simulink model "e03_MtrCtrl_MtrCtrl"  (R2024a)
settings: Solver=FixedStepDiscrete  StartTime=0.0  StopTime=1  FixedStep=mSim.dTime  MaxStep=Define.sModelSampleTime  RelTol=7.1420e-05
undefined symbols (not defined in the file): CnstCnst, CnstMde, CnstNr, E03CCTRL, E03INIT, E03LIM, E03MCMV, sTempGain
libraries: Lib_LPF x2
(part 1 of 3)
settings Model: Creator=user  LastModifiedBy=admin
settings SolverCC: MaxConsecutiveZCs=10000  ZeroCrossAlgorithm=Adaptive  AlgebraicLoopSolver=TrustRegion
settings DataIOCC: SaveOutput=off  DSMLogging=off  InspectSignalLogs=on  SaveTime=off  SignalLoggingName=logsout_Validator
settings OptimizationCC: BlockReduction=off  DefaultParameterBehavior=Inlined  UseDivisionForNetSlopeComputation=UseDivisionForReciprocalsOfIntegersOnly  GainParamInheritBuiltInType=on  UseFloatMulNetSlope=on  DefaultUnderspecifiedDataType=single  InlineInvariantSignals=on  BitwiseOrLogicalOp=Logical operator  PassReuseOutputArgsAs=Individual arguments  EfficientFloat2IntCast=on  LifeSpan=Inf  OptimizeBlockOrder=speed  DifferentSizesBufferReuse=on  EfficientTunableParamExpr=on
settings DebuggingCC: SignalInfNanChecking=error  SignalRangeChecking=error  ReadBeforeWriteMsg=EnableAllAsError  WriteAfterWriteMsg=EnableAllAsError  WriteAfterReadMsg=EnableAllAsError  AlgebraicLoopMsg=error  ArtificialAlgebraicLoopMsg=error  SaveWithDisabledLinksMsg=error  SaveWithParameterizedLinksMsg=error  BlockPriorityViolationMsg=error  SolverPrmCheckMsg=error  InheritedTsInSrcMsg=error  SingleTaskRateTransMsg=error  TasksWithSamePriorityMsg=error  SigSpecEnsureSampleTimeMsg=error  CheckMatrixSingularityMsg=error  IntegerOverflowMsg=error  ParameterUnderflowMsg=error  ParameterPrecisionLossMsg=error  ParameterTunabilityLossMsg=error  UnderSpecifiedDataTypeMsg=error  UnnecessaryDatatypeConvMsg=warning  VectorMatrixConversionMsg=error  SignalLabelMismatchMsg=error  UnconnectedInputMsg=error  UnconnectedOutputMsg=error  UnconnectedLineMsg=error  SFcnCompatibilityMsg=error  UniqueDataStoreMsg=error  BusObjectLabelMismatch=error  RootOutportRequireBusObject=error  AssertControl=DisableAll  ModelReferenceIOMismatchMessage=error  UnknownTsInhSupMsg=error  ModelReferenceDataLoggingMessage=error  ModelReferenceSymbolNameMessage=none  StateNameClashWarn=warning  StrictBusMsg=ErrorOnBusTreatedAsVector  NonBusSignalsTreatedAsBus=error  SFInvalidInputDataAccessInChartInitDiag=error  SFTransitionOutsideNaturalParentDiag=error  SFUnreachableExecutionPathDiag=error  SFUndirectedBroadcastEventsDiag=error  SFTransitionActionBeforeConditionDiag=error  SFTemporalDelaySmallerThanSampleTimeDiag=error  SFSelfTransitionDiag=error  SFExecutionAtInitializationDiag=error  IntegerSaturationMsg=error  UnitsInconsistencyMsg=none  VariantConditionMismatch=error
settings HardwareCC: ProdBitPerChar=16  ProdBitPerInt=16  ProdBitPerPointer=32  ProdBitPerSizeT=32  ProdBitPerPtrDiffT=32  ProdLargestAtomicInteger=Integer  ProdLargestAtomicFloat=None  ProdWordSize=16  ProdLongLongMode=on  ProdHWDeviceType=Texas Instruments->C2000
settings ModelReferenceCC: EnableRefExpFcnMdlSchedulingChecks=on  ModelReferenceNumInstancesAllowed=Single
settings SFSimCC: SimUseLocalCustomCode=off  CompileTimeRecursionLimit=0  EnableRuntimeRecursion=off  MATLABDynamicMemAlloc=off  CustomCodeUndefinedFunction=UseInterfaceOnly
settings RTWCC: Description=Embedded Coder  SystemTargetFile=ert.tlc  GenCodeOnly=on  TemplateMakefile=ert_default_tmf  GenerateReport=on  RTWUseLocalCustomCode=off  BuildConfiguration=Faster Runs  IncludeHyperlinkInReport=on  LaunchReport=on  GenerateTraceInfo=on  GenerateTraceReport=on  GenerateTraceReportSl=on  GenerateTraceReportSf=on  GenerateWebview=on  GenerateCodeMetricsReport=on  GenerateCodeReplacementReport=on  GPUComputeCapability=3.5  DLArmComputeVersion=19.05
settings CodeAppCC: ForceParamTrailComments=on  IgnoreCustomStorageClasses=off  MATLABFcnDesc=on  MangleLength=4  CustomSymbolStrGlobalVar=GvE03$N$M  CustomSymbolStrType=StrE03$N$M  CustomSymbolStrFcn=$N$M$F  CustomSymbolStrMacro=$N$M  DefineNamingRule=UpperCase  ParamNamingRule=UpperCase  SimulinkBlockComments=off  MATLABSourceComments=on  EnableCustomComments=on  ReqsInCode=on
settings ERTTargetCC: TargetLangStandard=C99 (ISO)  UtilityFuncGeneration=Shared location  MultiwordLength=2048  IncludeMdlTerminateFcn=off  CombineSignalStateStructs=on  SuppressErrorStatus=on  SupportAbsoluteTime=off  SupportNonFinite=off  ParenthesesLevel=Maximum  CastingMode=Standards  GenerateSharedConstants=off  InlinedParameterPlacement=NonHierarchical  ERTSrcFileBannerTemplate=t_code_template.cgt  ERTHdrFileBannerTemplate=t_code_template.cgt  ERTDataSrcFileTemplate=t_code_template.cgt  ERTDataHdrFileTemplate=t_code_template.cgt  ERTCustomFileTemplate=example_file_process.tlc  ERTFilePackagingFormat=CompactWithDataFile  PreserveExpressionOrder=on  SuppressUnreachableDefaultCases=off  EnableSignedLeftShifts=off  EnableSignedRightShifts=off  IndentStyle=Allman  IndentSize=4
settings ConfigComp: CovSaveName=coveragedata  CovMetricSettings=we  CovEnableCumulative=off  CovSaveCumulativeToWorkspaceVar=on  CovSaveSingleToWorkspaceVar=on  CovOutputDir=sldv_output/$ModelName$\sldv_covoutput  PSVerificationMode=BugFinder  PSModelRefIgnoreList=[]  PSEnableModelRefIgnoreList=off  PSModelRefMinMaxVerif=CheckAndConstrain  PSAutoStubLUT=on  DVModelCoverageObjectives=MCDC  DVTestSuiteOptimization=CombinedObjectives (Nonlinear Extended)  DVRebuildModelRepresentation=Always
settings SimscapeCC: SimscapeNormalizeSystem=off

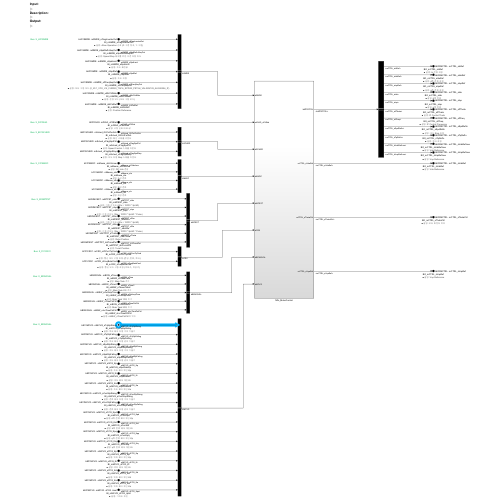
[thumbnail: Simulink's stored preview of the top-level diagram]
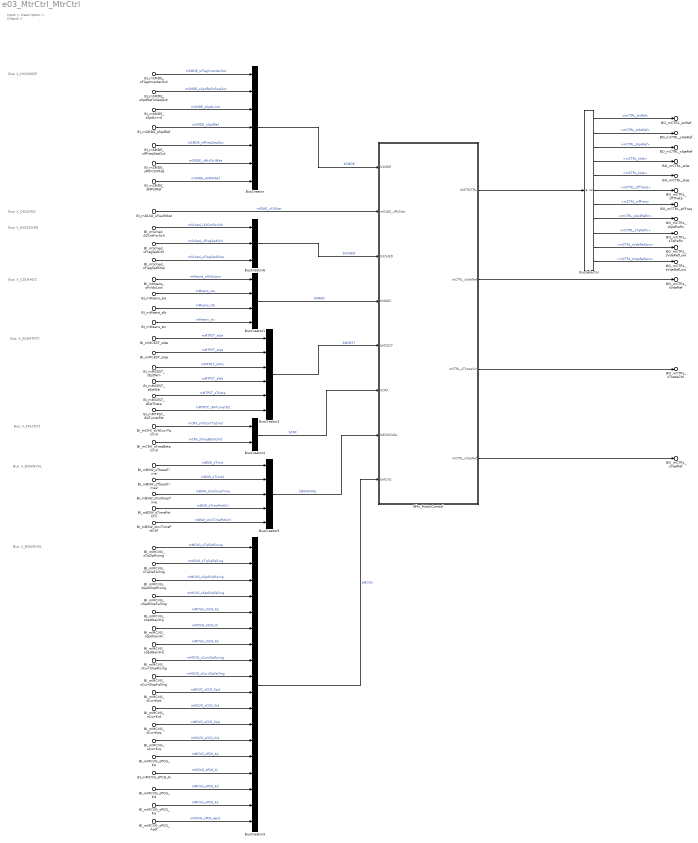
== system e03_MtrCtrl_MtrCtrl ==
  note: Bus: X_H01SMDE
  note: Input:
      | ▷
      | Description:
      | ▷
      | Output:
      | ▷
  note: Bus: X_D01DIAG
  note: Bus: X_B01SCHED
  note: Bus: X_C01MADC
  note: Bus: X_E02MTPST
  note: Bus: X_F01CRX1
  note: Bus: X_BSWGVAL
  note: Bus: X_BSWGVAL
  BI_mMsens_sIa : Inport  Description=■ 설명: A상 전류  PortName=bC01MADC  Element=mMsens_sIa
      settings: AttributesFormatString=%<Description>
  BI_mMsens_sIb : Inport  Description=■ 설명: B상 전류  PortName=bC01MADC  Element=mMsens_sIb
      settings: AttributesFormatString=%<Description>
  BI_mMsens_sIc : Inport  Description=■ 설명: C상 전류  PortName=bC01MADC  Element=mMsens_sIc
      settings: AttributesFormatString=%<Description>
  BI_mMsens_sHVdcLow : Inport  Description=■ 설명: DC Link 전압  PortName=bC01MADC  Element=mMsens_sHVdcLow
      settings: AttributesFormatString=%<Description>
  BI_mSched_uFlagSpdCtrl : Inport  Description=■ 설명: Speed Control 스케쥴 카운터  Port=2  PortName=bB01SCHED  Element=mSched_uFlagSpdCtrl
      settings: AttributesFormatString=%<Description>
  BI_mSched_uFlagSpdSlop : Inport  Description=■ 설명: 속도 지령 Slop 스케쥴 카운터  Port=2  PortName=bB01SCHED  Element=mSched_uFlagSpdSlop
      settings: AttributesFormatString=%<Description>
  BI_mSched_i32CntForSch : Inport  Description=■ 설명: 메인 스케쥴 카운터  Port=2  PortName=bB01SCHED  Element=mSched_i32CntForSch
      settings: AttributesFormatString=%<Description>
  BI_mBSW_sTbaseTime : Inport  Description=■ 설명: Main Task 주기  Port=3  PortName=bBSWGVAL  Element=mBSW_sTime
      settings: AttributesFormatString=%<Description>
  BI_mBSW_sTbaseTime2 : Inport  Description=■ 설명: Main Task 2배 주기  Port=3  PortName=bBSWGVAL  Element=mBSW_sTime2
      settings: AttributesFormatString=%<Description>
  BI_mBSW_sOutloopTime : Inport  Description=■ 설명: Main Task 10배 주기  Port=3  PortName=bBSWGVAL  Element=mBSW_sOutloopTime
      settings: AttributesFormatString=%<Description>
  BI_mBSW_sTimePstCtrl : Inport  Description=■ 설명: Main Task 30배 주기  Port=3  PortName=bBSWGVAL  Element=mBSW_sTimePstCtrl
      settings: AttributesFormatString=%<Description>
  BI_mBSW_sInvTimePstCtrl : Inport  Description=■ 설명: mBSW_sTimePstCtrl의 역수  Port=3  PortName=bBSWGVAL  Element=mBSW_sInvTimePstCtrl
      settings: AttributesFormatString=%<Description>
  BI_mMCVG_sPCG_Kp : Inport  Description=■ 설명: 위치 제어 게인 Kp  Port=4  PortName=bE01MCVG  Element=mMCVG_sPCG_Kp
      settings: AttributesFormatString=%<Description>
  BI_mMCVG_sPCG_Ki : Inport  Description=■ 설명: 위치 제어 게인 Ki  Port=4  PortName=bE01MCVG  Element=mMCVG_sPCG_Ki
      settings: AttributesFormatString=%<Description>
  BI_mMCVG_sPCG_Kd : Inport  Description=■ 설명: 위치 제어 게인 Kd  Port=4  PortName=bE01MCVG  Element=mMCVG_sPCG_Kd
      settings: AttributesFormatString=%<Description>
  BI_mMCVG_sPCG_Ka : Inport  Description=■ 설명: 위치 제어 게인 Ka  Port=4  PortName=bE01MCVG  Element=mMCVG_sPCG_Ka
      settings: AttributesFormatString=%<Description>
  BI_mMCVG_sPCG_Apst : Inport  Description=■ 설명: 가속도 게인  Port=4  PortName=bE01MCVG  Element=mMCVG_sPCG_Apst
      settings: AttributesFormatString=%<Description>
  BI_mMCVG_sSpdGainKp : Inport  Description=■ 설명: 속도 제어 게인 Kp  Port=4  PortName=bE01MCVG  Element=mMCVG_sSCG_Kp
      settings: AttributesFormatString=%<Description>
  BI_mMCVG_sSpdGainKi : Inport  Description=■ 설명: 속도 제어 게인 Ki  Port=4  PortName=bE01MCVG  Element=mMCVG_sSCG_Ki
      settings: AttributesFormatString=%<Description>
  BI_mMCVG_sSpdGainKa : Inport  Description=■ 설명: 속도 제어 게인 Ka  Port=4  PortName=bE01MCVG  Element=mMCVG_sSCG_Ka
      settings: AttributesFormatString=%<Description>
  BI_mMCVG_sCurrKpd : Inport  Description=■ 설명: d축 전류 제어 게인 Kp  Port=4  PortName=bE01MCVG  Element=mMCVG_sCCG_Kpd
      settings: AttributesFormatString=%<Description>
  BI_mMCVG_sCurrKid : Inport  Description=■ 설명: d축 전류 제어 게인 Ki  Port=4  PortName=bE01MCVG  Element=mMCVG_sCCG_Kid
      settings: AttributesFormatString=%<Description>
  BI_mMCVG_sCurrKpq : Inport  Description=■ 설명: q축 전류 제어 게인 Kp  Port=4  PortName=bE01MCVG  Element=mMCVG_sCCG_Kpq
      settings: AttributesFormatString=%<Description>
  BI_mMCVG_sCurrKiq : Inport  Description=■ 설명: q축 전류 제어 게인 Ki  Port=4  PortName=bE01MCVG  Element=mMCVG_sCCG_Kiq
      settings: AttributesFormatString=%<Description>
  BI_mMCVG_sSpdSlopRising : Inport  Description=■ 설명: 속도 제어 지령 가속 기울기  Port=4  PortName=bE01MCVG  Element=mMCVG_sSpdSlpRising
      settings: AttributesFormatString=%<Description>
  BI_mMCVG_sSpdSlopFalling : Inport  Description=■ 설명: 속도 제어 지령 감속 기울기  Port=4  PortName=bE01MCVG  Element=mMCVG_sSpdSlpFalling
      settings: AttributesFormatString=%<Description>
  BI_mMCVG_sTqSlpRising : Inport  Description=■ 설명: 토크 제어 지령 가속 기울기  Port=4  PortName=bE01MCVG  Element=mMCVG_sTqSlpRising
      settings: AttributesFormatString=%<Description>
  BI_mMCVG_sTqSlpFalling : Inport  Description=■ 설명: 토크 제어 지령 감속 기울기  Port=4  PortName=bE01MCVG  Element=mMCVG_sTqSlpFalling
      settings: AttributesFormatString=%<Description>
  BI_mMCVG_sCurrSlopRising : Inport  Description=■ 설명: 전류 제어 지령 가속 기울기  Port=4  PortName=bE01MCVG  Element=mMCVG_sCurrSlpRising
      settings: AttributesFormatString=%<Description>
  BI_mMCVG_sCurrSlopFalling : Inport  Description=■ 설명: 전류 제어 지령 감속 기울기  Port=4  PortName=bE01MCVG  Element=mMCVG_sCurrSlpFalling
      settings: AttributesFormatString=%<Description>
  BI_mDIAG_uFaultStat : Inport  Description=■ 설명: 고장 신호 대표 값  Port=5  PortName=bD01DIAG  Element=mDIAG_uFltStat
      settings: AttributesFormatString=%<Description>
  BI_mCRX_sVltCurrTqCmd : Inport  Description=■ 설명: 통신 모드 구동 지령 (전압, 전류, 토크)  Port=6  PortName=bF01CRX1  Element=mCRX_sVltCurrTqCmd
      settings: AttributesFormatString=%<Description>
  BI_mCRX_sFreqBetaCmd : Inport  Description=■ 설명: 통신 모드 구동 지령 (주파수, 위상각)  Port=6  PortName=bF01CRX1  Element=mCRX_sFreqBetaCmd
      settings: AttributesFormatString=%<Description>
  BI_mMCEST_sEstWm : Inport  Description=■ 설명: 기계 각속도 (Wm = 12000 * 2pi/60)  Port=7  PortName=bE02MCEST  Element=mMTPST_sWm
      settings: AttributesFormatString=%<Description>
  BI_mMCEST_sEstWe : Inport  Description=■ 설명: 기계 각속도 (We = 10000 * 2pi/60 * Poles)  Port=7  PortName=bE02MCEST  Element=mMTPST_sWe
      settings: AttributesFormatString=%<Description>
  BI_mMCEST_sEstTheta : Inport  Description=■ 설명: Rotor Position  Port=7  PortName=bE02MCEST  Element=mMTPST_sTheta
      settings: AttributesFormatString=%<Description>
  BI_mMTPST_i64TurretPst : Inport  Description=■ 설명: Turret Position  Port=7  PortName=bE02MCEST  Element=mMTPST_i64TurretPst
      settings: AttributesFormatString=%<Description>
  BI_mMCEST_sIde : Inport  Description=■ 설명: 기계 각속도 (Wm = 12000 * 2pi/60)  Port=7  PortName=bE02MCEST  Element=mMTPST_sIde
      settings: AttributesFormatString=%<Description>
  BI_mMCEST_sIqe : Inport  Description=■ 설명: 기계 각속도 (We = 10000 * 2pi/60 * Poles)  Port=7  PortName=bE02MCEST  Element=mMTPST_sIqe
      settings: AttributesFormatString=%<Description>
  BI_mSMDE_uFlagInverterOut : Inport  Description=■ 설명: Allow Operation 신호 (0: 구정 정지, 1: 구동)  Port=8  PortName=bH01SMDE  Element=mSMDE_uFlagInverterOut
      settings: AttributesFormatString=%<Description>
  BI_mSMDE_sSpdRefInSeqOut : Inport  Description=■ 설명: Speed Slop 제어를 위한 이전 지령 속도  Port=8  PortName=bH01SMDE  Element=mSMDE_sSpdRefInSeqOut
      settings: AttributesFormatString=%<Description>
  BI_mSMDE_sSpdLimit : Inport  Description=■ 설명: 속도 제한값  Port=8  PortName=bH01SMDE  Element=mSMDE_sSpdLimit
      settings: AttributesFormatString=%<Description>
  BI_mSMDE_sSpdRef : Inport  Description=■ 설명: 속도 지령  Port=8  PortName=bH01SMDE  Element=mSMDE_sSpdRef
      settings: AttributesFormatString=%<Description>
  BI_mSMDE_sIfFreqSeqOut : Inport  Description=■ 설명: 모터 구동 모드 (0_IO/1_VF/2_V/4_CURR/8_TQ/16_SPD/32_PST/64_VALIGN/128_ALIGN/256_IF)  Port=8  PortName=bH01SMDE  Element=mSMDE_sIfFreqSeqOut
      settings: AttributesFormatString=%<Description>
  BI_mSMDE_uMtrCtrlMde : Inport  Description=■ 설명: 운영 모드 (모터 구동 모드)  Port=8  PortName=bH01SMDE  Element=mSMDE_uMtrCtrlMde
      settings: AttributesFormatString=%<Description>
  BI_mSMDE_i64PstRef : Inport  Description=■ 설명: Position Reference  Port=8  PortName=bH01SMDE  Element=mSMDE_i64PstRef
      settings: AttributesFormatString=%<Description>
  BusCreator : BusCreator  Inputs=7
  BusCreator1 : BusCreator  Inputs=4
  BusCreator2 : BusCreator  Inputs=6
  BusCreator3 : BusCreator  Inputs=18
  BusCreator4 : BusCreator  Inputs=2
  BusCreator5 : BusCreator  Inputs=5
  BusCreator6 : BusCreator  Inputs=3
  BusSelector : BusSelector  OutputSignals=mCTRL_sIsRef,bCurrRefSelOut.mCTRL_sIdeRef,bCurrRefSelOut.mCTRL_sIqeRef,bCurrRefSelOut.mCTRL_sIde,bCurrRefSelOut.mCTRL_sIqe,mCTRL_sIfTheta,mCTRL_sIfFreq,mCTRL_sSpdRefIn,mCTRL_sTqRefIn,mCTRL_sVdeRefLow,mCTRL_sVqeRefLow
  Nftn_MotorControl : Subsystem
  BO_mCTRL_sIsRef : Outport  Description=■ 설명: Is 전류 지령  PortName=bE03MCTRL  Element=mCTRL_sIsRef
      settings: AttributesFormatString=%<Description>
  BO_mCTRL_sIdeRef : Outport  Description=■ 설명: d축 전류 지령  PortName=bE03MCTRL  Element=mCTRL_sIdeRef
      settings: AttributesFormatString=%<Description>
  BO_mCTRL_sIqeRef : Outport  Description=■ 설명: q축 전류 지령  PortName=bE03MCTRL  Element=mCTRL_sIqeRef
      settings: AttributesFormatString=%<Description>
  BO_mCTRL_sIde : Outport  Description=■ 설명: d축 전류  PortName=bE03MCTRL  Element=mCTRL_sIde
      settings: AttributesFormatString=%<Description>
  BO_mCTRL_sIqe : Outport  Description=■ 설명: q축 전류  PortName=bE03MCTRL  Element=mCTRL_sIqe
      settings: AttributesFormatString=%<Description>
  BO_mCTRL_sIfTheta : Outport  Description=■ 설명: IF Control Theta  PortName=bE03MCTRL  Element=mCTRL_sIfTheta
      settings: AttributesFormatString=%<Description>
  BO_mCTRL_sIfFreq : Outport  Description=■ 설명: IF Control Frequency  PortName=bE03MCTRL  Element=mCTRL_sIfFreq
      settings: AttributesFormatString=%<Description>
  BO_mCTRL_sSpdRefIn : Outport  Description=■ 설명: 속도 Slop 지령  PortName=bE03MCTRL  Element=mCTRL_sSpdRefIn
      settings: AttributesFormatString=%<Description>
  BO_mCTRL_sTqRefIn : Outport  Description=■ 설명: 토크 지령  PortName=bE03MCTRL  Element=mCTRL_sTqRefIn
      settings: AttributesFormatString=%<Description>
  BO_mCTRL_sVdeRefLow : Outport  Description=■ 설명: Vde Reference  PortName=bE03MCTRL  Element=mCTRL_sVdeRefLow
      settings: AttributesFormatString=%<Description>
  BO_mCTRL_sVqeRefLow : Outport  Description=■ 설명: Vqe Reference  PortName=bE03MCTRL  Element=mCTRL_sVqeRefLow
      settings: AttributesFormatString=%<Description>
  BO_mCTRL_sVdeRef : Outport  Description=■ 설명: Vde Reference  PortName=bE03MCTRL  Element=mCTRL_sVdeRef
      settings: AttributesFormatString=%<Description>
  BO_mCTRL_sVqeRef : Outport  Description=■ 설명: Vqe Reference  PortName=bE03MCTRL  Element=mCTRL_sVqeRef
      settings: AttributesFormatString=%<Description>
  BO_mCTRL_sThetaCtrl : Outport  Description=■ 설명: 모터 회전자 위치  PortName=bE03MCTRL  Element=mCTRL_sThetaCtrl
      settings: AttributesFormatString=%<Description>
  wires:
  BI_mBSW_sTbaseTime2/1 -> BusCreator5/2  "mBSW_sTime2"
  BusCreator5/1 -> Nftn_MotorControl/7(bBSWGVAL)  "bBSWGVAL"
  BI_mMCVG_sCurrKiq/1 -> BusCreator3/13  "mMCVG_sCCG_Kiq"
  BI_mMCVG_sSpdSlopRising/1 -> BusCreator3/3  "mMCVG_sSpdSlpRising"
  Nftn_MotorControl/1(bMTRCTRL) -> BusSelector/1
  BusSelector/1 -> BO_mCTRL_sIsRef/1  "<mCTRL_sIsRef>"
  BusCreator3/1 -> Nftn_MotorControl/8(bMCVG)  "bMCVG"
  BI_mMCVG_sSpdGainKa/1 -> BusCreator3/7  "mMCVG_sSCG_Ka"
  BI_mMCEST_sEstWe/1 -> BusCreator2/4  "mMTPST_sWe"
  BusSelector/2 -> BO_mCTRL_sIdeRef/1  "<mCTRL_sIdeRef>"
  BusCreator6/1 -> Nftn_MotorControl/3(bSCHED)  "bSCHED"
  BusCreator/1 -> Nftn_MotorControl/1(bSMDE)  "bSMDE"
  BI_mCRX_sFreqBetaCmd/1 -> BusCreator4/2  "mCRX_sFreqBetaCmd"
  BusSelector/7 -> BO_mCTRL_sIfFreq/1  "<mCTRL_sIfFreq>"
  BI_mDIAG_uFaultStat/1 -> Nftn_MotorControl/2(mDIAG_uFltStat)  "mDIAG_uFltStat"
  BI_mBSW_sOutloopTime/1 -> BusCreator5/3  "mBSW_sOutloopTime"
  BusSelector/3 -> BO_mCTRL_sIqeRef/1  "<mCTRL_sIqeRef>"
  BusSelector/10 -> BO_mCTRL_sVdeRefLow/1  "<mCTRL_sVdeRefLow>"
  BI_mMsens_sIc/1 -> BusCreator1/4  "mMsens_sIc"
  BI_mSched_uFlagSpdCtrl/1 -> BusCreator6/2  "mSched_uFlagSpdCtrl"
  BI_mMsens_sIa/1 -> BusCreator1/2  "mMsens_sIa"
  BusSelector/8 -> BO_mCTRL_sSpdRefIn/1  "<mCTRL_sSpdRefIn>"
  BI_mSMDE_sSpdRef/1 -> BusCreator/4  "mSMDE_sSpdRef"
  BusSelector/4 -> BO_mCTRL_sIde/1  "<mCTRL_sIde>"
  BI_mSched_uFlagSpdSlop/1 -> BusCreator6/3  "mSched_uFlagSpdSlop"
  BI_mMsens_sIb/1 -> BusCreator1/3  "mMsens_sIb"
  Nftn_MotorControl/3(mCTRL_sThetaCtrl) -> BO_mCTRL_sThetaCtrl/1
  BusSelector/11 -> BO_mCTRL_sVqeRefLow/1  "<mCTRL_sVqeRefLow>"
  BusSelector/9 -> BO_mCTRL_sTqRefIn/1  "<mCTRL_sTqRefIn>"
  BI_mMCEST_sIqe/1 -> BusCreator2/2  "mMTPST_sIqe"
  Nftn_MotorControl/2(mCTRL_sVdeRef) -> BO_mCTRL_sVdeRef/1
  BI_mMCVG_sCurrSlopRising/1 -> BusCreator3/8  "mMCVG_sCurrSlpRising"
  BI_mSMDE_sSpdRefInSeqOut/1 -> BusCreator/2  "mSMDE_sSpdRefInSeqOut"
  BI_mMCEST_sEstTheta/1 -> BusCreator2/5  "mMTPST_sTheta"
  BusCreator4/1 -> Nftn_MotorControl/6(bCRX)  "bCRX"
  BusSelector/6 -> BO_mCTRL_sIfTheta/1  "<mCTRL_sIfTheta>"
  BusSelector/5 -> BO_mCTRL_sIqe/1  "<mCTRL_sIqe>"
  Nftn_MotorControl/4(mCTRL_sVqeRef) -> BO_mCTRL_sVqeRef/1
  BI_mBSW_sTbaseTime/1 -> BusCreator5/1  "mBSW_sTime"
  BI_mMCVG_sSpdGainKp/1 -> BusCreator3/5  "mMCVG_sSCG_Kp"
  BI_mMCVG_sSpdGainKi/1 -> BusCreator3/6  "mMCVG_sSCG_Ki"
  BI_mMCVG_sSpdSlopFalling/1 -> BusCreator3/4  "mMCVG_sSpdSlpFalling"
  BI_mMCVG_sCurrKpq/1 -> BusCreator3/12  "mMCVG_sCCG_Kpq"
  BI_mSched_i32CntForSch/1 -> BusCreator6/1  "mSched_i32CntForSch"
  BI_mSMDE_sIfFreqSeqOut/1 -> BusCreator/5  "mSMDE_sIfFreqSeqOut"
  BusCreator1/1 -> Nftn_MotorControl/4(bMADC)  "bMADC"
  BI_mMCVG_sCurrSlopFalling/1 -> BusCreator3/9  "mMCVG_sCurrSlpFalling"
  BusCreator2/1 -> Nftn_MotorControl/5(bMCEST)  "bMCEST"
  BI_mMCVG_sCurrKpd/1 -> BusCreator3/10  "mMCVG_sCCG_Kpd"
  BI_mSMDE_uFlagInverterOut/1 -> BusCreator/1  "mSMDE_uFlagInverterOut"
  BI_mMCVG_sCurrKid/1 -> BusCreator3/11  "mMCVG_sCCG_Kid"
  BI_mMCEST_sEstWm/1 -> BusCreator2/3  "mMTPST_sWm"
  BI_mMsens_sHVdcLow/1 -> BusCreator1/1  "mMsens_sHVdcLow"
  BI_mSMDE_uMtrCtrlMde/1 -> BusCreator/6  "mSMDE_uMtrCtrlMde"
  BI_mMCEST_sIde/1 -> BusCreator2/1  "mMTPST_sIde"
  BI_mCRX_sVltCurrTqCmd/1 -> BusCreator4/1  "mCRX_sVltCurrTqCmd"
  BI_mMCVG_sTqSlpRising/1 -> BusCreator3/1  "mMCVG_sTqSlpRising"
  BI_mMCVG_sTqSlpFalling/1 -> BusCreator3/2  "mMCVG_sTqSlpFalling"
  BI_mMCVG_sPCG_Kp/1 -> BusCreator3/14  "mMCVG_sPCG_Kp"
  BI_mMCVG_sPCG_Ki/1 -> BusCreator3/15  "mMCVG_sPCG_Ki"
  BI_mMCVG_sPCG_Kd/1 -> BusCreator3/16  "mMCVG_sPCG_Kd"
  BI_mMCVG_sPCG_Ka/1 -> BusCreator3/17  "mMCVG_sPCG_Ka"
  BI_mMCVG_sPCG_Apst/1 -> BusCreator3/18  "mMCVG_sPCG_Apst"
  BI_mBSW_sTimePstCtrl/1 -> BusCreator5/4  "mBSW_sTimePstCtrl"
  BI_mSMDE_i64PstRef/1 -> BusCreator/7  "mSMDE_i64PstRef"
  BI_mMTPST_i64TurretPst/1 -> BusCreator2/6  "mMTPST_i64TurretPst"
  BI_mBSW_sInvTimePstCtrl/1 -> BusCreator5/5  "mBSW_sInvTimePstCtrl"
  BI_mSMDE_sSpdLimit/1 -> BusCreator/3  "mSMDE_sSpdLimit"

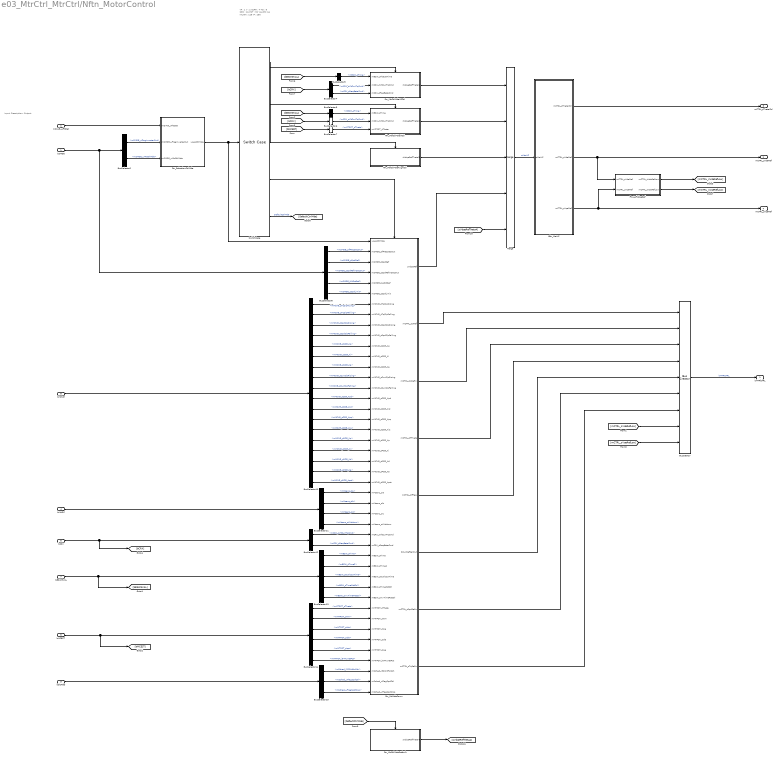
== system e03_MtrCtrl_MtrCtrl/Nftn_MotorControl ==
  note: VF : 1
      | V : 2
      | CURR : 4
      | TQ : 8
      | SPD : 16
      | PST : 32
      | VALIGN: 64
      | IALIGN : 128
      | IF : 256
  note: Input:
      | Description:
      | Output:
  bSMDE : Inport
  mDIAG_uFltStat : Inport  Port=2
  bSCHED : Inport  Port=3
  bMADC : Inport  Port=4
  bMCEST : Inport  Port=5
  bCRX : Inport  Port=6
  bBSWGVAL : Inport  Port=7
  bMCVG : Inport  Port=8
  BusCreator : BusCreator  Inputs=9
  BusSelector10 : BusSelector  OutputSignals=mMCVG_sTqSlpRising,mMCVG_sTqSlpFalling,mMCVG_sSpdSlpRising,mMCVG_sSpdSlpFalling,mMCVG_sSCG_Kp,mMCVG_sSCG_Ki,mMCVG_sSCG_Ka,mMCVG_sCurrSlpRising,mMCVG_sCurrSlpFalling,mMCVG_sCCG_Kpd,mMCVG_sCCG_Kid,mMCVG_sCCG_Kpq,mMCVG_sCCG_Kiq,mMCVG_sPCG_Kp,mMCVG_sPCG_Ki,mMCVG_sPCG_Kd,mMCVG_sPCG_Ka,mMCVG_sPCG_Apst
  BusSelector11 : BusSelector  OutputSignals=mMsens_sIa,mMsens_sIb,mMsens_sIc,mMsens_sHVdcLow
  BusSelector12 : BusSelector  OutputSignals=mCRX_sVltCurrTqCmd,mCRX_sFreqBetaCmd
  BusSelector13 : BusSelector  OutputSignals=mBSW_sTime,mBSW_sTime2,mBSW_sOutloopTime,mBSW_sTimePstCtrl,mBSW_sInvTimePstCtrl
  BusSelector14 : BusSelector  OutputSignals=mMTPST_sTheta,mMTPST_sWm,mMTPST_sWe,mMTPST_sIde,mMTPST_sIqe,mMTPST_i64TurretPst
  BusSelector15 : BusSelector  OutputSignals=mSched_i32CntForSch,mSched_uFlagSpdCtrl,mSched_uFlagSpdSlop
  BusSelector2 : BusSelector  OutputSignals=mSMDE_uFlagInverterOut,mSMDE_uMtrCtrlMde
  BusSelector3 : BusSelector  OutputSignals=mBSW_sTime
  BusSelector4 : BusSelector  OutputSignals=mCRX_sVltCurrTqCmd,mCRX_sFreqBetaCmd
  BusSelector5 : BusSelector  OutputSignals=mBSW_sTime
  BusSelector6 : BusSelector  OutputSignals=mCRX_sVltCurrTqCmd
  BusSelector7 : BusSelector  OutputSignals=mMTPST_sTheta
  BusSelector8 : BusSelector  OutputSignals=mSMDE_sIfFreqSeqOut,mSMDE_sSpdRef,mSMDE_sSpdRefInSeqOut,mSMDE_i64PstRef,mSMDE_sSpdLimit
  Ftn_LpfVdqeRef : Subsystem  TreatAsAtomicUnit=on
      settings: RTWSystemCode=Nonreusable function  RTWFcnNameOpts=Use subsystem name
  Ftn_MtrCtrlMdeAlignCtrl : Subsystem
      settings: RTWSystemCode=Nonreusable function  RTWFcnNameOpts=Use subsystem name
  Ftn_MtrCtrlMdeDefault : Subsystem
      settings: RTWSystemCode=Nonreusable function  RTWFcnNameOpts=Use subsystem name
  Ftn_MtrCtrlMdeVCtrl : Subsystem
      settings: RTWSystemCode=Nonreusable function  RTWFcnNameOpts=Use subsystem name
  Ftn_MtrCtrlMdeVFCtrl : Subsystem
      settings: RTWSystemCode=Nonreusable function  RTWFcnNameOpts=Use subsystem name
  Ftn_MtrMdeComn : Subsystem  RTWFileName=Motor_Control
      settings: RTWSystemCode=Nonreusable function  RTWFcnNameOpts=Use subsystem name
  Ftn_SelectionCtrlMde : Subsystem  TreatAsAtomicUnit=on
      settings: RTWSystemCode=Nonreusable function  RTWFcnNameOpts=Use subsystem name
  Merge : Merge  Tag=PWMOUT  Description=|  Inputs=5
      | mVe.Ve_Ref_d
      | mVe.Ve_Ref_q
      | mTheta.App_sin
      | mTheta.App_cos
  Nftn_MerVC : Subsystem
  SwitchCase : SwitchCase  CaseConditions="{1, 2, 64, [4, 8, 16, 32, 128,  256]}"
  bMTRCTRL : Outport
  mCTRL_sVdeRef : Outport  Description=■ 설명: Vde Reference  Port=2  OutMin=-1000  OutMax=1000
      settings: AttributesFormatString=%<Description>
  mCTRL_sThetaCtrl : Outport  Description=■ 설명: Rotor Position  Port=3  OutMin=0  OutMax=6.2832
      settings: AttributesFormatString=%<Description>
  mCTRL_sVqeRef : Outport  Description=■ 설명: Vqe Reference  Port=4  OutMin=-1000  OutMax=1000
      settings: AttributesFormatString=%<Description>
  wires:
  Ftn_MtrMdeComn/6(bCurrRefSelOut) -> BusCreator/5
  Ftn_MtrMdeComn/4(mCTRL_sIfTheta) -> BusCreator/3
  Ftn_MtrMdeComn/5(mCTRL_sIfFreq) -> BusCreator/4
  Ftn_MtrMdeComn/2(mCTRL_sIsRef) -> BusCreator/1
  Ftn_MtrMdeComn/3(mCTRL_sIsRefIn) -> BusCreator/2
  bBSWGVAL/1 -> [bBSWGVAL], BusSelector13/1
  Ftn_SelectionCtrlMde/1(uAppCtrlMde) -> SwitchCase/1, Ftn_MtrMdeComn/1(uAppCtrlMde)
  SwitchCase/5 -> [DefaultCtrlMde]  "DefaultCtrlMde"
  [bBSWGVAL] -> BusSelector3/1
  bCRX/1 -> [bCRX], BusSelector12/1
  bMCEST/1 -> [bMCEST], BusSelector14/1
  [bCRX] -> BusSelector4/1
  Merge/1 -> Nftn_MerVC/1(aMerVC)  "aMerVC"
  Nftn_MerVC/1(mCTRL_sThetaCtrl) -> mCTRL_sThetaCtrl/1
  Ftn_MtrMdeComn/7(mCTRL_sSpdRefIn) -> BusCreator/6
  Ftn_MtrMdeComn/8(mCTRL_sTqRefIn) -> BusCreator/7
  [DefaultCtrlMde] -> Ftn_MtrCtrlMdeDefault/Action
  SwitchCase/4 -> Ftn_MtrMdeComn/Action
  SwitchCase/3 -> Ftn_MtrCtrlMdeAlignCtrl/Action
  SwitchCase/2 -> Ftn_MtrCtrlMdeVCtrl/Action
  SwitchCase/1 -> Ftn_MtrCtrlMdeVFCtrl/Action
  Ftn_MtrMdeComn/1(sVdqeRef) -> Merge/4
  Ftn_MtrCtrlMdeVFCtrl/1(sVdqeRefTheta1) -> Merge/1
  Ftn_MtrCtrlMdeVCtrl/1(sVdqeRefTheta2) -> Merge/2
  Ftn_MtrCtrlMdeAlignCtrl/1(sVdqeRefTheta3) -> Merge/3
  Ftn_MtrCtrlMdeDefault/1(sVdqeRefTheta4) -> [sVdqeRefTheta4]
  [sVdqeRefTheta4] -> Merge/5
  [mCTRL_sVqeRefLow] -> BusCreator/9
  [mCTRL_sVdeRefLow] -> BusCreator/8
  BusCreator/1 -> bMTRCTRL/1  "bMTRCTRL"
  Nftn_MerVC/2(mCTRL_sVdeRef) -> Ftn_LpfVdqeRef/1(mCTRL_sVdeRef), mCTRL_sVdeRef/1
  Nftn_MerVC/3(mCTRL_sVqeRef) -> Ftn_LpfVdqeRef/2(mCTRL_sVqeRef), mCTRL_sVqeRef/1
  Ftn_LpfVdqeRef/1(mCTRL_sVdeRefLow) -> [mCTRL_sVdeRefLow]
  Ftn_LpfVdqeRef/2(mCTRL_sVqeRefLow) -> [mCTRL_sVqeRefLow]
  BusSelector3/1 -> Ftn_MtrCtrlMdeVFCtrl/1(mBSW_sTbaseTime)  "<mBSW_sTime>"
  BusSelector4/1 -> Ftn_MtrCtrlMdeVFCtrl/2(mCRX_sVltCurrTqCmd)  "<mCRX_sVltCurrTqCmd>"
  BusSelector4/2 -> Ftn_MtrCtrlMdeVFCtrl/3(mCRX_sFreqBetaCmd)  "<mCRX_sFreqBetaCmd>"
  bSMDE/1 -> BusSelector2/1, BusSelector8/1
  BusSelector2/1 -> Ftn_SelectionCtrlMde/2(mSMDE_uFlagInverterOut)  "<mSMDE_uFlagInverterOut>"
  BusSelector2/2 -> Ftn_SelectionCtrlMde/3(mSMDE_uMtrCtrlMde)  "<mSMDE_uMtrCtrlMde>"
  mDIAG_uFltStat/1 -> Ftn_SelectionCtrlMde/1(mDIAG_uFltStat)
  BusSelector5/1 -> Ftn_MtrCtrlMdeVCtrl/1(mBSW_sTime)  "<mBSW_sTime>"
  [bBSWGVAL] -> BusSelector5/1
  BusSelector6/1 -> Ftn_MtrCtrlMdeVCtrl/2(mCRX_sVltCurrTqCmd)  "<mCRX_sVltCurrTqCmd>"
  [bCRX] -> BusSelector6/1
  BusSelector7/1 -> Ftn_MtrCtrlMdeVCtrl/3(mMTPST_sTheta)  "<mMTPST_sTheta>"
  [bMCEST] -> BusSelector7/1
  BusSelector8/1 -> Ftn_MtrMdeComn/2(mSMDE_sIfFreqSeqOut)  "<mSMDE_sIfFreqSeqOut>"
  BusSelector8/2 -> Ftn_MtrMdeComn/3(mSMDE_sSpdRef)  "<mSMDE_sSpdRef>"
  BusSelector8/3 -> Ftn_MtrMdeComn/4(mSMDE_sSpdRefInSeqOut)  "<mSMDE_sSpdRefInSeqOut>"
  bMCVG/1 -> BusSelector10/1
  BusSelector11/2 -> Ftn_MtrMdeComn/26(mMsens_sIb)  "<mMsens_sIb>"
  BusSelector11/3 -> Ftn_MtrMdeComn/27(mMsens_sIc)  "<mMsens_sIc>"
  BusSelector11/1 -> Ftn_MtrMdeComn/25(mMsens_sIa)  "<mMsens_sIa>"
  bMADC/1 -> BusSelector11/1
  BusSelector11/4 -> Ftn_MtrMdeComn/28(mMsens_sHVdcLow)  "<mMsens_sHVdcLow>"
  BusSelector12/1 -> Ftn_MtrMdeComn/29(mCRX_sVltCurrTqCmd)  "<mCRX_sVltCurrTqCmd>"
  BusSelector12/2 -> Ftn_MtrMdeComn/30(mCRX_sFreqBetaCmd)  "<mCRX_sFreqBetaCmd>"
  BusSelector13/1 -> Ftn_MtrMdeComn/31(mBSW_sTime)  "<mBSW_sTime>"
  BusSelector13/2 -> Ftn_MtrMdeComn/32(mBSW_sTime2)  "<mBSW_sTime2>"
  BusSelector13/3 -> Ftn_MtrMdeComn/33(mBSW_sOutloopTime)  "<mBSW_sOutloopTime>"
  BusSelector14/1 -> Ftn_MtrMdeComn/36(mMTPST_sTheta)  "<mMTPST_sTheta>"
  BusSelector14/2 -> Ftn_MtrMdeComn/37(mMTPST_sWm)  "<mMTPST_sWm>"
  BusSelector14/3 -> Ftn_MtrMdeComn/38(mMTPST_sWe)  "<mMTPST_sWe>"
  BusSelector14/4 -> Ftn_MtrMdeComn/39(mMTPST_sIde)  "<mMTPST_sIde>"
  BusSelector14/5 -> Ftn_MtrMdeComn/40(mMTPST_sIqe)  "<mMTPST_sIqe>"
  BusSelector15/3 -> Ftn_MtrMdeComn/44(mSched_uFlagSpdSlop)  "<mSched_uFlagSpdSlop>"
  BusSelector15/2 -> Ftn_MtrMdeComn/43(mSched_uFlagSpdCtrl)  "<mSched_uFlagSpdCtrl>"
  bSCHED/1 -> BusSelector15/1
  BusSelector10/1 -> Ftn_MtrMdeComn/7(mMCVG_sTqSlpRising)  "<mMCVG_sTqSlpRising>"
  BusSelector10/2 -> Ftn_MtrMdeComn/8(mMCVG_sTqSlpFalling)  "<mMCVG_sTqSlpFalling>"
  BusSelector10/3 -> Ftn_MtrMdeComn/9(mMCVG_sSpdSlpRising)  "<mMCVG_sSpdSlpRising>"
  BusSelector10/4 -> Ftn_MtrMdeComn/10(mMCVG_sSpdSlpFalling)  "<mMCVG_sSpdSlpFalling>"
  BusSelector10/5 -> Ftn_MtrMdeComn/11(mMCVG_sSCG_Kp)  "<mMCVG_sSCG_Kp>"
  BusSelector10/6 -> Ftn_MtrMdeComn/12(mMCVG_sSCG_Ki)  "<mMCVG_sSCG_Ki>"
  BusSelector10/7 -> Ftn_MtrMdeComn/13(mMCVG_sSCG_Ka)  "<mMCVG_sSCG_Ka>"
  BusSelector10/8 -> Ftn_MtrMdeComn/14(mMCVG_sCurrSlpRising)  "<mMCVG_sCurrSlpRising>"
  BusSelector10/9 -> Ftn_MtrMdeComn/15(mMCVG_sCurrSlpFalling)  "<mMCVG_sCurrSlpFalling>"
  BusSelector10/10 -> Ftn_MtrMdeComn/16(mMCVG_sCCG_Kpd)  "<mMCVG_sCCG_Kpd>"
  BusSelector10/11 -> Ftn_MtrMdeComn/17(mMCVG_sCCG_Kid)  "<mMCVG_sCCG_Kid>"
  BusSelector10/12 -> Ftn_MtrMdeComn/18(mMCVG_sCCG_Kpq)  "<mMCVG_sCCG_Kpq>"
  BusSelector10/13 -> Ftn_MtrMdeComn/19(mMCVG_sCCG_Kiq)  "<mMCVG_sCCG_Kiq>"
  BusSelector10/14 -> Ftn_MtrMdeComn/20(mMCVG_sPCG_Kp)  "<mMCVG_sPCG_Kp>"
  BusSelector10/15 -> Ftn_MtrMdeComn/21(mMCVG_sPCG_Ki)  "<mMCVG_sPCG_Ki>"
  BusSelector10/16 -> Ftn_MtrMdeComn/22(mMCVG_sPCG_Kd)  "<mMCVG_sPCG_Kd>"
  BusSelector10/17 -> Ftn_MtrMdeComn/23(mMCVG_sPCG_Ka)  "<mMCVG_sPCG_Ka>"
  BusSelector10/18 -> Ftn_MtrMdeComn/24(mMCVG_sPCG_Apst)  "<mMCVG_sPCG_Apst>"
  BusSelector13/4 -> Ftn_MtrMdeComn/34(mBSW_sTimePstCtrl)  "<mBSW_sTimePstCtrl>"
  BusSelector15/1 -> Ftn_MtrMdeComn/42(mSched_i32CntForSch)  "<mSched_i32CntForSch>"
  BusSelector8/4 -> Ftn_MtrMdeComn/5(mSMDE_i64PstRef)  "<mSMDE_i64PstRef>"
  BusSelector14/6 -> Ftn_MtrMdeComn/41(mMTPST_i64TurretPst)  "<mMTPST_i64TurretPst>"
  BusSelector13/5 -> Ftn_MtrMdeComn/35(mBSW_sInvTimePstCtrl)  "<mBSW_sInvTimePstCtrl>"
  BusSelector8/5 -> Ftn_MtrMdeComn/6(mSMDE_sSpdLimit)  "<mSMDE_sSpdLimit>"

== system e03_MtrCtrl_MtrCtrl/Nftn_MotorControl/Ftn_LpfVdqeRef ==
  note: Input:
      | Description:
      | Output:
  mCTRL_sVdeRef : Inport  Description=■ 설명: Vde Reference  OutMin=-1000  OutMax=1000
      settings: AttributesFormatString=%<Description>
  mCTRL_sVqeRef : Inport  Description=■ 설명: Vqe Reference  Port=2  OutMin=-1000  OutMax=1000
      settings: AttributesFormatString=%<Description>
  LowPassFilter : Lib_LPF/LowPassFilter  La=E03MTRSWF.sVdqeLa  Lb=E03MTRSWF.sVdqeLb  Init_Value=0
  LowPassFilter1 : Lib_LPF/LowPassFilter  La=E03MTRSWF.sVdqeLa  Lb=E03MTRSWF.sVdqeLb  Init_Value=0
  mCTRL_sVdeRefLow : Outport  Description=■ 설명: Vde Reference (필터 후)  OutMin=-1000  OutMax=1000
      settings: AttributesFormatString=%<Description>
  mCTRL_sVqeRefLow : Outport  Description=■ 설명: Vqe Reference (필터 후)  Port=2  OutMin=-1000  OutMax=1000
      settings: AttributesFormatString=%<Description>
  wires:
  mCTRL_sVqeRef/1 -> LowPassFilter/1
  mCTRL_sVdeRef/1 -> LowPassFilter1/1
  LowPassFilter/1 -> mCTRL_sVqeRefLow/1  "mCTRL_sVqeRefLow"
  LowPassFilter1/1 -> mCTRL_sVdeRefLow/1  "mCTRL_sVdeRefLow"

== system e03_MtrCtrl_MtrCtrl/Nftn_MotorControl/Ftn_MtrCtrlMdeAlignCtrl ==
  note: Input:
      | Description:
      | Output:
  ActionPort : ActionPort  ActionPortLabel=case [ 64 ]:
  CB_C_PI2_INV_360 : Constant  Value=CnstCnst.C_PI2_INV_360
  CB_E03MCMV_sAlign16Angle : Constant  Value=E03MCMV.sAlign16Angle
  CB_E03MCMV_sAlign16Vout : Constant  Value=E03MCMV.sAlign16Vout
  CB_sAlignVdeRef : Constant  Value=0  OutDataTypeStr=single
  Mux : Mux  Inputs=3
  Product : Product
  sVdqeRefTheta3 : Outport  Description=|  OutMin=-1000  OutMax=1000  VectorParamsAs1DForOutWhenUnconnected=off
      | ■ 설명: 제어 모드 전류 출력 Mux 신호
      | -.[0] : d축 전압 지령
      | -.[1] : q축 전압 지령
      | -.[2] : Theta control cmd (270deg)
      settings: AttributesFormatString=%<Description>
  wires:
  Mux/1 -> sVdqeRefTheta3/1  "sVdqeRefTheta3"
  CB_sAlignVdeRef/1 -> Mux/1  "sAlignVdeRef"
  Product/1 -> Mux/3  "sAlignTheta"
  CB_C_PI2_INV_360/1 -> Product/2  "C_PI2_INV_360"
  CB_E03MCMV_sAlign16Angle/1 -> Product/1  "sAlign16Angle"
  CB_E03MCMV_sAlign16Vout/1 -> Mux/2  "sAlignVqeRef"

== system e03_MtrCtrl_MtrCtrl/Nftn_MotorControl/Ftn_MtrCtrlMdeDefault ==
  note: Input:
      | Description:
      | Output:
  ActionPort : ActionPort  ActionPortLabel=default:
  CB_sThetaCtrlDefaultMde : Constant  Value=0  OutDataTypeStr=single
  CB_sVdeRefDefaultMde : Constant  Value=0  OutDataTypeStr=single
  CB_sVqeRefDefaultMde : Constant  Value=0  OutDataTypeStr=single
  Mux : Mux  Inputs=3
  sVdqeRefTheta4 : Outport  Description=|  OutMin=-1000  OutMax=1000  VectorParamsAs1DForOutWhenUnconnected=off
      | ■ 설명: 제어 출력 Mux 신호
      | -. [0] : d축 전압 지령
      | -. [1] : q축 전압 지령
      | -. [2] : Theta control cmd
      settings: AttributesFormatString=%<Description>
  wires:
  CB_sVqeRefDefaultMde/1 -> Mux/2  "sVqeRefDefaultMde"
  CB_sThetaCtrlDefaultMde/1 -> Mux/3  "sThetaCtrlDefaultMde"
  CB_sVdeRefDefaultMde/1 -> Mux/1  "sVdeRefDefaultMde"
  Mux/1 -> sVdqeRefTheta4/1  "sVdqeRefTheta4"

== system e03_MtrCtrl_MtrCtrl/Nftn_MotorControl/Ftn_MtrCtrlMdeVCtrl ==
  note: Input:
      | Description:
      | Output:
  mBSW_sTime : Inport  Description=■ 설명: 주기, sTime (1/14kH)  OutMin=0  OutMax=0.0000714286
      settings: AttributesFormatString=%<Description>
  mCRX_sVltCurrTqCmd : Inport  Description=■ 설명: uVltCurrTqCmd(Voltage / Current / Torque Reference)  Port=2  OutMin=-398.3  OutMax=398.3
      settings: AttributesFormatString=%<Description>
  mMTPST_sTheta : Inport  Description=■ 설명: Rotor Position  Port=3  OutMin=0  OutMax=6.2832
      settings: AttributesFormatString=%<Description>
  ActionPort : ActionPort  ActionPortLabel=case [ 2 ]:
  Ftn_VCtrlSlop : Subsystem  TreatAsAtomicUnit=on
      settings: RTWSystemCode=Nonreusable function  RTWFcnNameOpts=Use subsystem name
  Nftn_MuxVCtrl : Subsystem
  sVdqeRefTheta2 : Outport  Description=|  OutMin=-1000  OutMax=1000  VectorParamsAs1DForOutWhenUnconnected=off
      | ■ 설명: 제어 모드 전류 출력 Mux 신호
      | -.[0] : d축 전압 지령
      | -.[1] : q축 전압 지령
      | -.[2] : Theta control cmd
      settings: AttributesFormatString=%<Description>
  wires:
  Nftn_MuxVCtrl/1(sVdqeRefTheta2) -> sVdqeRefTheta2/1
  Ftn_VCtrlSlop/1(sVVqeRef) -> Nftn_MuxVCtrl/1(sVqeRef_V)
  mBSW_sTime/1 -> Ftn_VCtrlSlop/2(mBSW_sTime)
  mCRX_sVltCurrTqCmd/1 -> Ftn_VCtrlSlop/1(mCRX_sVltCurrTqCmd)
  mMTPST_sTheta/1 -> Nftn_MuxVCtrl/2(mMTPST_sTheta)

== system e03_MtrCtrl_MtrCtrl/Nftn_MotorControl/Ftn_MtrCtrlMdeVFCtrl ==
  note: Input:
      | Description:
      | Output:
  mBSW_sTbaseTime : Inport  Description=■ 설명: 주기, sTime (1/10kH)  OutMin=0  OutMax=0.0000714286
      settings: AttributesFormatString=%<Description>
  mCRX_sVltCurrTqCmd : Inport  Description=■ 설명: uVltCurrTqCmd(Voltage / Current / Torque Reference)  Port=2  OutMin=-398.3  OutMax=398.3
      settings: AttributesFormatString=%<Description>
  mCRX_sFreqBetaCmd : Inport  Description=■ 설명: uFreqBetaCmd(Frequency / Beta Reference)  Port=3  OutMin=0  OutMax=409.5
      settings: AttributesFormatString=%<Description>
  ActionPort : ActionPort  ActionPortLabel=case [ 1 ]:
  Ftn_VfCtrlSlop : Subsystem  TreatAsAtomicUnit=on
      settings: RTWSystemCode=Nonreusable function  RTWFcnNameOpts=Use subsystem name
  Nftn_MuxVFCtrl : Subsystem
  sVdqeRefTheta1 : Outport  Description=|  OutMin=-1000  OutMax=1000  VectorParamsAs1DForOutWhenUnconnected=off
      | ■ 설명: 제어 모드 전류 출력 Mux 신호
      | -.[0] : d축 전압 지령
      | -.[1] : q축 전압 지령
      | -.[2] : Theta control cmd
      settings: AttributesFormatString=%<Description>
  wires:
  mCRX_sFreqBetaCmd/1 -> Nftn_MuxVFCtrl/1(mCRX_sFreqBetaCmd)
  Ftn_VfCtrlSlop/1(sVfVqeRef) -> Nftn_MuxVFCtrl/2(sVfVqeRef)
  Nftn_MuxVFCtrl/1(sVdqeRefTheta1) -> sVdqeRefTheta1/1
  mBSW_sTbaseTime/1 -> Nftn_MuxVFCtrl/3(mBSW_sTime), Ftn_VfCtrlSlop/2(mBSW_sTime)
  mCRX_sVltCurrTqCmd/1 -> Ftn_VfCtrlSlop/1(mCRX_sVltCurrTqCmd)
